simulink model "test2"  (R2016a)
settings: Solver=FixedStepDiscrete  StartTime=0.0  StopTime=10.0  RelTol=1e-3
libraries: arduinolib x6
settings Model: SimulationMode=external  ExtModeTrigDuration=2  Creator=shohei  LastModifiedBy=shohei
settings OptimizationCC: OptimizeModelRefInitCode=on  LifeSpan=1  MaxStackSize=64
settings HardwareCC: ProdBitPerInt=16  ProdBitPerPointer=16  ProdLargestAtomicFloat=None  ProdWordSize=8  ProdHWDeviceType=Atmel->AVR
settings RTWCC: SystemTargetFile=ert.tlc  HardwareBoard=Arduino Uno  TemplateMakefile=ert_default_tmf  GenerateReport=on  Toolchain=Arduino AVR v1.6.1  BuildConfiguration=Faster Runs  IncludeHyperlinkInReport=on  LaunchReport=on  GenerateTraceInfo=on  GenerateTraceReport=on  GenerateTraceReportSl=on  GenerateTraceReportSf=on  GenerateTraceReportEml=on
settings CodeAppCC: ForceParamTrailComments=on  IgnoreCustomStorageClasses=off  OperatorAnnotations=on  SimulinkDataObjDesc=on  SFDataObjDesc=on  MATLABFcnDesc=on  InsertBlockDesc=on  MATLABSourceComments=on
settings ERTTargetCC: SupportContinuousTime=on  SupportVariableSizeSignals=on

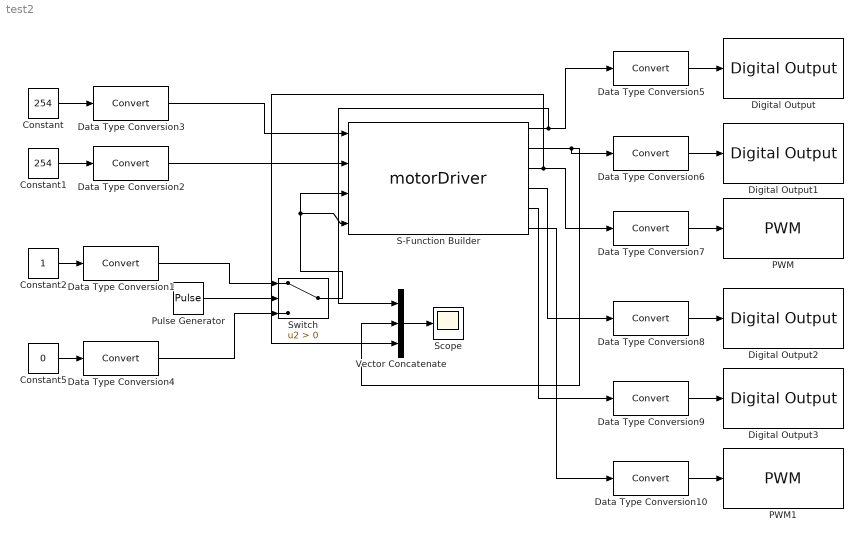
== system test2 ==
  Constant : Constant  Value=254
  Constant1 : Constant  Value=254
  Constant2 : Constant
  Constant5 : Constant  Value=0
  Data Type Conversion{1..10} (10 alike) : DataTypeConversion
  Digital Output : arduinolib/Digital Output  pinNumber=4  blockPlatform=arduino
  Digital Output1 : arduinolib/Digital Output  pinNumber=5  blockPlatform=arduino
  Digital Output2 : arduinolib/Digital Output  pinNumber=7  blockPlatform=arduino
  Digital Output3 : arduinolib/Digital Output  pinNumber=8  blockPlatform=arduino
  PWM : arduinolib/PWM  pinNumber=6  blockPlatform=arduino
  PWM1 : arduinolib/PWM  pinNumber=9  blockPlatform=arduino
  Pulse Generator : DiscretePulseGenerator  PulseType=Time based  Period=4  PulseWidth=50
  S-Function Builder : S-Function  InitFcn=try, set_param(gcb,'FunctionName','motorDriver'), end  FunctionName=motorDriver  SFunctionModules=motorDriver_wrapper  SFunctionDeploymentMode=off  EnableBusSupport=off  mask(S-Function Builder){}
      mask help: Simulink:masks:SFunctionBuilder_MD
      mask init:
      | val = [[.9  0.75 0.75 1 1 .9 .9 1]',[1 1 0.75 0.75 .9 .9 1 .9]'];try , sys = get_param(gcb,'SfunBuilderFcnName');if isempty(sys), sys = get_param(gcb,'FunctionName'); end,catch, sys = get_param(gcb,'FunctionName'); end
      settings: CopyFcn=set_param(gcbh,'LinkStatus','none')  PreSaveFcn=try, set_param(gcb,'FunctionName','motorDriver'), end  OpenFcn=sfunctionwizard(gcbh)
      mask Display: plot(val(:,1),val(:,2)),disp(sys), port_label('input',1,'speed1'), port_label('input',2,'speed2'), port_label('input',3,'direction1'), port_label('input',4,'direction2'), port_label('output',1,'m1_1'), port_label('output',2,'m1_2'), port_label('output',3,'m1_pwm'), port_label('output',4,'m2_1'), port_label('output',5,'m2_2'), port_label('output',6,'m2_pwm')
  Scope : Scope
  Switch : Switch  Criteria=u2 > Threshold
  Vector Concatenate : Concatenate  NumInputs=3
  wires:
  Constant/1 -> Data Type Conversion3/1
  Constant1/1 -> Data Type Conversion2/1
  Constant2/1 -> Data Type Conversion1/1
  Data Type Conversion3/1 -> S-Function Builder/1
  Data Type Conversion2/1 -> S-Function Builder/2
  Data Type Conversion1/1 -> Switch/1
  Pulse Generator/1 -> Switch/2
  Data Type Conversion4/1 -> Switch/3
  Constant5/1 -> Data Type Conversion4/1
  Switch/1 -> S-Function Builder/3, S-Function Builder/4
  Data Type Conversion5/1 -> Digital Output/1
  Data Type Conversion6/1 -> Digital Output1/1
  Data Type Conversion7/1 -> PWM/1
  Data Type Conversion8/1 -> Digital Output2/1
  Data Type Conversion9/1 -> Digital Output3/1
  Data Type Conversion10/1 -> PWM1/1
  S-Function Builder/1 -> Vector Concatenate/1, Data Type Conversion5/1
  S-Function Builder/2 -> Vector Concatenate/2, Data Type Conversion6/1
  S-Function Builder/3 -> Vector Concatenate/3, Data Type Conversion7/1
  S-Function Builder/4 -> Data Type Conversion8/1
  S-Function Builder/5 -> Data Type Conversion9/1
  S-Function Builder/6 -> Data Type Conversion10/1
  Vector Concatenate/1 -> Scope/1
